simulink model "window_and_fft_test"  (R2012b)
settings: Solver=ode45  StartTime=0.0  StopTime=100000  RelTol=1e-3
values from neighbouring files (symbols this model uses):
  Fs = 640e6    (= 640000000)    [filter_coefficients.m]    (also in filter_design.m; filter_design_getting_order.m)
undefined symbols (not defined in the file or in its folder): get, pfb_coeff_gen_calc, sided, Two, xlipgetpartsetting
undefined symbols (not defined in the file): A_cos, A_sin, B_cos, B_sin, C_cos, C_sin, casper_coef, D_cos, D_sin
libraries: xbsIndex_r4 x7054, casper_library_misc x43, casper_library_delays x25, dspsnks4 x18, dspspect3 x8, dspsigops x4, xps_library x2, xbsReplacements_r4 x2, casper_library_pfbs x2, simulink x1
(part 4 of 85)

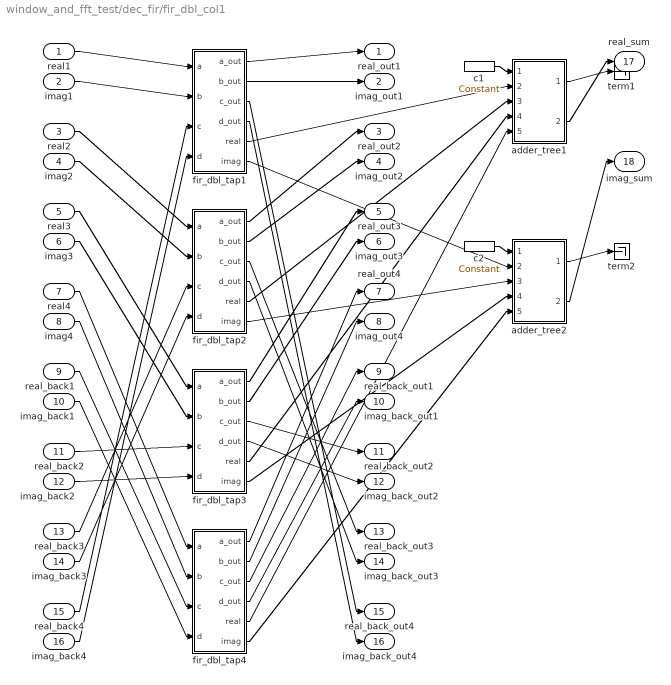
== system window_and_fft_test/dec_fir/fir_dbl_col1 ==
  real1 : Inport
  imag1 : Inport  Port=2
  real2 : Inport  Port=3
  imag2 : Inport  Port=4
  real3 : Inport  Port=5
  imag3 : Inport  Port=6
  real4 : Inport  Port=7
  imag4 : Inport  Port=8
  real_back1 : Inport  Port=9
  imag_back1 : Inport  Port=10
  real_back2 : Inport  Port=11
  imag_back2 : Inport  Port=12
  real_back3 : Inport  Port=13
  imag_back3 : Inport  Port=14
  real_back4 : Inport  Port=15
  imag_back4 : Inport  Port=16
  adder_tree1 : Subsystem  AncestorBlock=casper_library_misc/adder_tree  mask(adder_tree){n_inputs=4, latency=1, adder_imp=DSP48, first_stage_hdl=on}
      mask prompts: n_inputs "Number of Inputs"; latency "Add Latency"; adder_imp "Adder implementation"; first_stage_hdl "Use behavioural HDL for first stage of adders"
      mask help:
      | Sums all inputs using a tree of adds and delays.
      |
      | Number of inputs: The number of inputs to the block to be summed
      | Add latency: The number of clock cycles to perform one addition (affects timing)..
      | Adder implementation: choice of fabric or DSP48E core, or behavioral HDL
      | Use behavioural HDL for first stage of adders: Causes the first stage of adders to be absorbed into DSP blocks if multipliers precede them (Virtex 5). Overrides Adder implementation
      mask init:
      | adder_tree_init(gcb, ...
      |     'n_inputs', n_inputs, ...
      |     'latency', latency, ...
      |     'adder_imp', adder_imp, ...
      |     'first_stage_hdl', first_stage_hdl);
      settings: AttributesFormatString=latency 2
      mask Help: eval('xlWeb(''http://casper.berkeley.edu/wiki/Adder_tree'')')
      mask TypeOptions adder_imp: Behavioral | Fabric | DSP48
  adder_tree2 : Subsystem  AncestorBlock=casper_library_misc/adder_tree  mask(adder_tree){n_inputs=4, latency=1, adder_imp=DSP48, first_stage_hdl=on}
      mask prompts: n_inputs "Number of Inputs"; latency "Add Latency"; adder_imp "Adder implementation"; first_stage_hdl "Use behavioural HDL for first stage of adders"
      mask help:
      | Sums all inputs using a tree of adds and delays.
      |
      | Number of inputs: The number of inputs to the block to be summed
      | Add latency: The number of clock cycles to perform one addition (affects timing)..
      | Adder implementation: choice of fabric or DSP48E core, or behavioral HDL
      | Use behavioural HDL for first stage of adders: Causes the first stage of adders to be absorbed into DSP blocks if multipliers precede them (Virtex 5). Overrides Adder implementation
      mask init:
      | adder_tree_init(gcb, ...
      |     'n_inputs', n_inputs, ...
      |     'latency', latency, ...
      |     'adder_imp', adder_imp, ...
      |     'first_stage_hdl', first_stage_hdl);
      settings: AttributesFormatString=latency 2
      mask Help: eval('xlWeb(''http://casper.berkeley.edu/wiki/Adder_tree'')')
      mask TypeOptions adder_imp: Behavioral | Fabric | DSP48
  c1 : xbsIndex_r4/Constant  const=1  gui_display_data_type=Fixed-point  arith_type=Signed (2's comp)  n_bits=16  bin_pt=14  preci_type=Single  exp_width=8  frac_width=24  explicit_period=on  period=1  equ=P=C  opselect=C  inp2=PCIN>>17  opr=+  inp1=P  carry=CIN  dbl_ovrd=off  block_type=constant
  c2 : xbsIndex_r4/Constant  const=1  gui_display_data_type=Fixed-point  arith_type=Signed (2's comp)  n_bits=16  bin_pt=14  preci_type=Single  exp_width=8  frac_width=24  explicit_period=on  period=1  equ=P=C  opselect=C  inp2=PCIN>>17  opr=+  inp1=P  carry=CIN  dbl_ovrd=off  block_type=constant
  fir_dbl_tap1 : Subsystem  AncestorBlock=casper_library_downconverter/fir_dbl_tap  mask(fir_dbl_tap){factor=0.037109, add_latency=add_latency, mult_latency=mult_latency, coeff_bit_width=coeff_bit_width, coeff_bin_pt=coeff_bin_pt}
      mask prompts: add_latency "Add latency"; mult_latency "Mult latency"; coeff_bit_width "Coefficient bit width"; coeff_bin_pt "Coefficient binary point"
      mask init:
      | fir_dbl_tap_init(gcb, ...
      |     'factor', factor, ...
      |     'add_latency', add_latency, ...
      |     'mult_latency', mult_latency, ...
      |     'coeff_bit_width', coeff_bit_width, ...
      |     'coeff_bin_pt', coeff_bin_pt);
      mask Help: eval('xlWeb(''http://casper.berkeley.edu/wiki/Fir_dbl_tap'')')
  fir_dbl_tap2 : Subsystem  AncestorBlock=casper_library_downconverter/fir_dbl_tap  mask(fir_dbl_tap){factor=0.023207, add_latency=add_latency, mult_latency=mult_latency, coeff_bit_width=coeff_bit_width, coeff_bin_pt=coeff_bin_pt}
      mask prompts: add_latency "Add latency"; mult_latency "Mult latency"; coeff_bit_width "Coefficient bit width"; coeff_bin_pt "Coefficient binary point"
      mask init: same as window_and_fft_test/dec_fir/fir_dbl_col1/fir_dbl_tap1
      mask Help: eval('xlWeb(''http://casper.berkeley.edu/wiki/Fir_dbl_tap'')')
  fir_dbl_tap3 : Subsystem  AncestorBlock=casper_library_downconverter/fir_dbl_tap  mask(fir_dbl_tap){factor=0.012354, add_latency=add_latency, mult_latency=mult_latency, coeff_bit_width=coeff_bit_width, coeff_bin_pt=coeff_bin_pt}
      mask prompts: add_latency "Add latency"; mult_latency "Mult latency"; coeff_bit_width "Coefficient bit width"; coeff_bin_pt "Coefficient binary point"
      mask init: same as window_and_fft_test/dec_fir/fir_dbl_col1/fir_dbl_tap1
      mask Help: eval('xlWeb(''http://casper.berkeley.edu/wiki/Fir_dbl_tap'')')
  fir_dbl_tap4 : Subsystem  AncestorBlock=casper_library_downconverter/fir_dbl_tap  mask(fir_dbl_tap){factor=0.0056253, add_latency=add_latency, mult_latency=mult_latency, coeff_bit_width=coeff_bit_width, coeff_bin_pt=coeff_bin_pt}
      mask prompts: add_latency "Add latency"; mult_latency "Mult latency"; coeff_bit_width "Coefficient bit width"; coeff_bin_pt "Coefficient binary point"
      mask init: same as window_and_fft_test/dec_fir/fir_dbl_col1/fir_dbl_tap1
      mask Help: eval('xlWeb(''http://casper.berkeley.edu/wiki/Fir_dbl_tap'')')
  term1 : Terminator
  term2 : Terminator
  real_out1 : Outport
  imag_out1 : Outport  Port=2
  real_out2 : Outport  Port=3
  imag_out2 : Outport  Port=4
  real_out3 : Outport  Port=5
  imag_out3 : Outport  Port=6
  real_out4 : Outport  Port=7
  imag_out4 : Outport  Port=8
  real_back_out1 : Outport  Port=9
  imag_back_out1 : Outport  Port=10
  real_back_out2 : Outport  Port=11
  imag_back_out2 : Outport  Port=12
  real_back_out3 : Outport  Port=13
  imag_back_out3 : Outport  Port=14
  real_back_out4 : Outport  Port=15
  imag_back_out4 : Outport  Port=16
  real_sum : Outport  Port=17
  imag_sum : Outport  Port=18
  wires:
  adder_tree1/1(sync_out) -> term1/1
  adder_tree2/1(sync_out) -> term2/1
  c1/1 -> adder_tree1/1(sync)
  c2/1 -> adder_tree2/1(sync)
  adder_tree1/2(dout) -> real_sum/1
  adder_tree2/2(dout) -> imag_sum/1
  real1/1 -> fir_dbl_tap1/1(a)
  imag1/1 -> fir_dbl_tap1/2(b)
  real_back4/1 -> fir_dbl_tap1/3(c)
  imag_back4/1 -> fir_dbl_tap1/4(d)
  fir_dbl_tap1/1(a_out) -> real_out1/1
  fir_dbl_tap1/2(b_out) -> imag_out1/1
  fir_dbl_tap1/3(c_out) -> real_back_out4/1
  fir_dbl_tap1/4(d_out) -> imag_back_out4/1
  fir_dbl_tap1/5(real) -> adder_tree1/2(din1)
  fir_dbl_tap1/6(imag) -> adder_tree2/2(din1)
  real2/1 -> fir_dbl_tap2/1(a)
  imag2/1 -> fir_dbl_tap2/2(b)
  real_back3/1 -> fir_dbl_tap2/3(c)
  imag_back3/1 -> fir_dbl_tap2/4(d)
  fir_dbl_tap2/1(a_out) -> real_out2/1
  fir_dbl_tap2/2(b_out) -> imag_out2/1
  fir_dbl_tap2/3(c_out) -> real_back_out3/1
  fir_dbl_tap2/4(d_out) -> imag_back_out3/1
  fir_dbl_tap2/5(real) -> adder_tree1/3(din2)
  fir_dbl_tap2/6(imag) -> adder_tree2/3(din2)
  real3/1 -> fir_dbl_tap3/1(a)
  imag3/1 -> fir_dbl_tap3/2(b)
  real_back2/1 -> fir_dbl_tap3/3(c)
  imag_back2/1 -> fir_dbl_tap3/4(d)
  fir_dbl_tap3/1(a_out) -> real_out3/1
  fir_dbl_tap3/2(b_out) -> imag_out3/1
  fir_dbl_tap3/3(c_out) -> real_back_out2/1
  fir_dbl_tap3/4(d_out) -> imag_back_out2/1
  fir_dbl_tap3/5(real) -> adder_tree1/4(din3)
  fir_dbl_tap3/6(imag) -> adder_tree2/4(din3)
  real4/1 -> fir_dbl_tap4/1(a)
  imag4/1 -> fir_dbl_tap4/2(b)
  real_back1/1 -> fir_dbl_tap4/3(c)
  imag_back1/1 -> fir_dbl_tap4/4(d)
  fir_dbl_tap4/1(a_out) -> real_out4/1
  fir_dbl_tap4/2(b_out) -> imag_out4/1
  fir_dbl_tap4/3(c_out) -> real_back_out1/1
  fir_dbl_tap4/4(d_out) -> imag_back_out1/1
  fir_dbl_tap4/5(real) -> adder_tree1/5(din4)
  fir_dbl_tap4/6(imag) -> adder_tree2/5(din4)

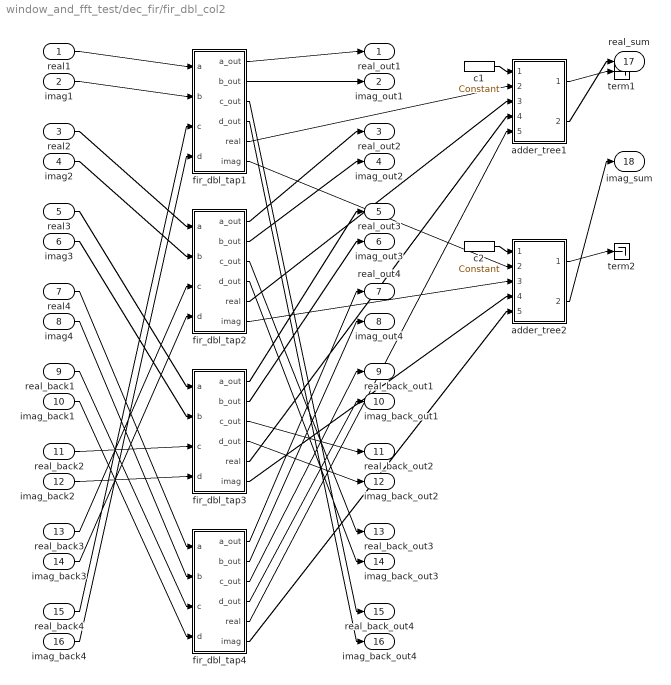
== system window_and_fft_test/dec_fir/fir_dbl_col2 ==
  real1 : Inport
  imag1 : Inport  Port=2
  real2 : Inport  Port=3
  imag2 : Inport  Port=4
  real3 : Inport  Port=5
  imag3 : Inport  Port=6
  real4 : Inport  Port=7
  imag4 : Inport  Port=8
  real_back1 : Inport  Port=9
  imag_back1 : Inport  Port=10
  real_back2 : Inport  Port=11
  imag_back2 : Inport  Port=12
  real_back3 : Inport  Port=13
  imag_back3 : Inport  Port=14
  real_back4 : Inport  Port=15
  imag_back4 : Inport  Port=16
  adder_tree1 : Subsystem  AncestorBlock=casper_library_misc/adder_tree  mask(adder_tree){n_inputs=4, latency=1, adder_imp=DSP48, first_stage_hdl=on}
      mask prompts: n_inputs "Number of Inputs"; latency "Add Latency"; adder_imp "Adder implementation"; first_stage_hdl "Use behavioural HDL for first stage of adders"
      mask help:
      | Sums all inputs using a tree of adds and delays.
      |
      | Number of inputs: The number of inputs to the block to be summed
      | Add latency: The number of clock cycles to perform one addition (affects timing)..
      | Adder implementation: choice of fabric or DSP48E core, or behavioral HDL
      | Use behavioural HDL for first stage of adders: Causes the first stage of adders to be absorbed into DSP blocks if multipliers precede them (Virtex 5). Overrides Adder implementation
      mask init:
      | adder_tree_init(gcb, ...
      |     'n_inputs', n_inputs, ...
      |     'latency', latency, ...
      |     'adder_imp', adder_imp, ...
      |     'first_stage_hdl', first_stage_hdl);
      settings: AttributesFormatString=latency 2
      mask Help: eval('xlWeb(''http://casper.berkeley.edu/wiki/Adder_tree'')')
      mask TypeOptions adder_imp: Behavioral | Fabric | DSP48
  adder_tree2 : Subsystem  AncestorBlock=casper_library_misc/adder_tree  mask(adder_tree){n_inputs=4, latency=1, adder_imp=DSP48, first_stage_hdl=on}
      mask prompts: n_inputs "Number of Inputs"; latency "Add Latency"; adder_imp "Adder implementation"; first_stage_hdl "Use behavioural HDL for first stage of adders"
      mask help:
      | Sums all inputs using a tree of adds and delays.
      |
      | Number of inputs: The number of inputs to the block to be summed
      | Add latency: The number of clock cycles to perform one addition (affects timing)..
      | Adder implementation: choice of fabric or DSP48E core, or behavioral HDL
      | Use behavioural HDL for first stage of adders: Causes the first stage of adders to be absorbed into DSP blocks if multipliers precede them (Virtex 5). Overrides Adder implementation
      mask init:
      | adder_tree_init(gcb, ...
      |     'n_inputs', n_inputs, ...
      |     'latency', latency, ...
      |     'adder_imp', adder_imp, ...
      |     'first_stage_hdl', first_stage_hdl);
      settings: AttributesFormatString=latency 2
      mask Help: eval('xlWeb(''http://casper.berkeley.edu/wiki/Adder_tree'')')
      mask TypeOptions adder_imp: Behavioral | Fabric | DSP48
  c1 : xbsIndex_r4/Constant  const=1  gui_display_data_type=Fixed-point  arith_type=Signed (2's comp)  n_bits=16  bin_pt=14  preci_type=Single  exp_width=8  frac_width=24  explicit_period=on  period=1  equ=P=C  opselect=C  inp2=PCIN>>17  opr=+  inp1=P  carry=CIN  dbl_ovrd=off  block_type=constant
  c2 : xbsIndex_r4/Constant  const=1  gui_display_data_type=Fixed-point  arith_type=Signed (2's comp)  n_bits=16  bin_pt=14  preci_type=Single  exp_width=8  frac_width=24  explicit_period=on  period=1  equ=P=C  opselect=C  inp2=PCIN>>17  opr=+  inp1=P  carry=CIN  dbl_ovrd=off  block_type=constant
  fir_dbl_tap1 : Subsystem  AncestorBlock=casper_library_downconverter/fir_dbl_tap  mask(fir_dbl_tap){factor=0.08556, add_latency=add_latency, mult_latency=mult_latency, coeff_bit_width=coeff_bit_width, coeff_bin_pt=coeff_bin_pt}
      mask prompts: add_latency "Add latency"; mult_latency "Mult latency"; coeff_bit_width "Coefficient bit width"; coeff_bin_pt "Coefficient binary point"
      mask init: same as window_and_fft_test/dec_fir/fir_dbl_col1/fir_dbl_tap1
      mask Help: eval('xlWeb(''http://casper.berkeley.edu/wiki/Fir_dbl_tap'')')
  fir_dbl_tap2 : Subsystem  AncestorBlock=casper_library_downconverter/fir_dbl_tap  mask(fir_dbl_tap){factor=0.079092, add_latency=add_latency, mult_latency=mult_latency, coeff_bit_width=coeff_bit_width, coeff_bin_pt=coeff_bin_pt}
      mask prompts: add_latency "Add latency"; mult_latency "Mult latency"; coeff_bit_width "Coefficient bit width"; coeff_bin_pt "Coefficient binary point"
      mask init: same as window_and_fft_test/dec_fir/fir_dbl_col1/fir_dbl_tap1
      mask Help: eval('xlWeb(''http://casper.berkeley.edu/wiki/Fir_dbl_tap'')')
  fir_dbl_tap3 : Subsystem  AncestorBlock=casper_library_downconverter/fir_dbl_tap  mask(fir_dbl_tap){factor=0.067391, add_latency=add_latency, mult_latency=mult_latency, coeff_bit_width=coeff_bit_width, coeff_bin_pt=coeff_bin_pt}
      mask prompts: add_latency "Add latency"; mult_latency "Mult latency"; coeff_bit_width "Coefficient bit width"; coeff_bin_pt "Coefficient binary point"
      mask init: same as window_and_fft_test/dec_fir/fir_dbl_col1/fir_dbl_tap1
      mask Help: eval('xlWeb(''http://casper.berkeley.edu/wiki/Fir_dbl_tap'')')
  fir_dbl_tap4 : Subsystem  AncestorBlock=casper_library_downconverter/fir_dbl_tap  mask(fir_dbl_tap){factor=0.052572, add_latency=add_latency, mult_latency=mult_latency, coeff_bit_width=coeff_bit_width, coeff_bin_pt=coeff_bin_pt}
      mask prompts: add_latency "Add latency"; mult_latency "Mult latency"; coeff_bit_width "Coefficient bit width"; coeff_bin_pt "Coefficient binary point"
      mask init: same as window_and_fft_test/dec_fir/fir_dbl_col1/fir_dbl_tap1
      mask Help: eval('xlWeb(''http://casper.berkeley.edu/wiki/Fir_dbl_tap'')')
  term1 : Terminator
  term2 : Terminator
  real_out1 : Outport
  imag_out1 : Outport  Port=2
  real_out2 : Outport  Port=3
  imag_out2 : Outport  Port=4
  real_out3 : Outport  Port=5
  imag_out3 : Outport  Port=6
  real_out4 : Outport  Port=7
  imag_out4 : Outport  Port=8
  real_back_out1 : Outport  Port=9
  imag_back_out1 : Outport  Port=10
  real_back_out2 : Outport  Port=11
  imag_back_out2 : Outport  Port=12
  real_back_out3 : Outport  Port=13
  imag_back_out3 : Outport  Port=14
  real_back_out4 : Outport  Port=15
  imag_back_out4 : Outport  Port=16
  real_sum : Outport  Port=17
  imag_sum : Outport  Port=18
  wires:
  adder_tree1/1(sync_out) -> term1/1
  adder_tree2/1(sync_out) -> term2/1
  c1/1 -> adder_tree1/1(sync)
  c2/1 -> adder_tree2/1(sync)
  adder_tree1/2(dout) -> real_sum/1
  adder_tree2/2(dout) -> imag_sum/1
  real1/1 -> fir_dbl_tap1/1(a)
  imag1/1 -> fir_dbl_tap1/2(b)
  real_back4/1 -> fir_dbl_tap1/3(c)
  imag_back4/1 -> fir_dbl_tap1/4(d)
  fir_dbl_tap1/1(a_out) -> real_out1/1
  fir_dbl_tap1/2(b_out) -> imag_out1/1
  fir_dbl_tap1/3(c_out) -> real_back_out4/1
  fir_dbl_tap1/4(d_out) -> imag_back_out4/1
  fir_dbl_tap1/5(real) -> adder_tree1/2(din1)
  fir_dbl_tap1/6(imag) -> adder_tree2/2(din1)
  real2/1 -> fir_dbl_tap2/1(a)
  imag2/1 -> fir_dbl_tap2/2(b)
  real_back3/1 -> fir_dbl_tap2/3(c)
  imag_back3/1 -> fir_dbl_tap2/4(d)
  fir_dbl_tap2/1(a_out) -> real_out2/1
  fir_dbl_tap2/2(b_out) -> imag_out2/1
  fir_dbl_tap2/3(c_out) -> real_back_out3/1
  fir_dbl_tap2/4(d_out) -> imag_back_out3/1
  fir_dbl_tap2/5(real) -> adder_tree1/3(din2)
  fir_dbl_tap2/6(imag) -> adder_tree2/3(din2)
  real3/1 -> fir_dbl_tap3/1(a)
  imag3/1 -> fir_dbl_tap3/2(b)
  real_back2/1 -> fir_dbl_tap3/3(c)
  imag_back2/1 -> fir_dbl_tap3/4(d)
  fir_dbl_tap3/1(a_out) -> real_out3/1
  fir_dbl_tap3/2(b_out) -> imag_out3/1
  fir_dbl_tap3/3(c_out) -> real_back_out2/1
  fir_dbl_tap3/4(d_out) -> imag_back_out2/1
  fir_dbl_tap3/5(real) -> adder_tree1/4(din3)
  fir_dbl_tap3/6(imag) -> adder_tree2/4(din3)
  real4/1 -> fir_dbl_tap4/1(a)
  imag4/1 -> fir_dbl_tap4/2(b)
  real_back1/1 -> fir_dbl_tap4/3(c)
  imag_back1/1 -> fir_dbl_tap4/4(d)
  fir_dbl_tap4/1(a_out) -> real_out4/1
  fir_dbl_tap4/2(b_out) -> imag_out4/1
  fir_dbl_tap4/3(c_out) -> real_back_out1/1
  fir_dbl_tap4/4(d_out) -> imag_back_out1/1
  fir_dbl_tap4/5(real) -> adder_tree1/5(din4)
  fir_dbl_tap4/6(imag) -> adder_tree2/5(din4)

== system window_and_fft_test/dec_fir/imag_sum ==
  sync : Inport
  din1 : Inport  Port=2
  din2 : Inport  Port=3
  addr1 : xbsIndex_r4/AddSub  mode=Addition  use_carryin=off  use_carryout=off  en=off  latency=1  precision=Full  arith_type=Unsigned  n_bits=16  bin_pt=14  quantization=Truncate  overflow=Wrap  dbl_ovrd=off  use_behavioral_HDL=off  hw_selection=DSP48  pipelined=on  use_rpm=on  block_type=addsub
  sync_delay : xbsIndex_r4/Delay  rst=off  infoeditControl=Selection of Reset will increase slice count due to use of real FFs and instead of SRLs  en=off  latency=1  dbl_ovrd=off  reg_retiming=on  block_type=delay
      settings: block_version=11.4
  sync_out : Outport
  dout : Outport  Port=2
  wires:
  sync/1 -> sync_delay/1
  sync_delay/1 -> sync_out/1
  din1/1 -> addr1/1
  din2/1 -> addr1/2
  addr1/1 -> dout/1

== system window_and_fft_test/dec_fir/real_sum ==
  sync : Inport
  din1 : Inport  Port=2
  din2 : Inport  Port=3
  addr1 : xbsIndex_r4/AddSub  mode=Addition  use_carryin=off  use_carryout=off  en=off  latency=1  precision=Full  arith_type=Unsigned  n_bits=16  bin_pt=14  quantization=Truncate  overflow=Wrap  dbl_ovrd=off  use_behavioral_HDL=off  hw_selection=DSP48  pipelined=on  use_rpm=on  block_type=addsub
  sync_delay : xbsIndex_r4/Delay  rst=off  infoeditControl=Selection of Reset will increase slice count due to use of real FFs and instead of SRLs  en=off  latency=1  dbl_ovrd=off  reg_retiming=on  block_type=delay
      settings: block_version=11.4
  sync_out : Outport
  dout : Outport  Port=2
  wires:
  sync/1 -> sync_delay/1
  sync_delay/1 -> sync_out/1
  din1/1 -> addr1/1
  din2/1 -> addr1/2
  addr1/1 -> dout/1

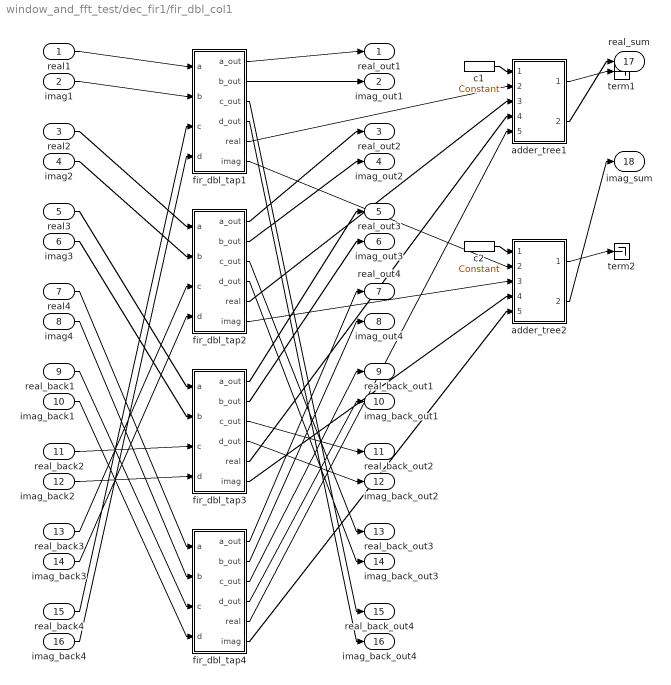
== system window_and_fft_test/dec_fir1/fir_dbl_col1 ==
  real1 : Inport
  imag1 : Inport  Port=2
  real2 : Inport  Port=3
  imag2 : Inport  Port=4
  real3 : Inport  Port=5
  imag3 : Inport  Port=6
  real4 : Inport  Port=7
  imag4 : Inport  Port=8
  real_back1 : Inport  Port=9
  imag_back1 : Inport  Port=10
  real_back2 : Inport  Port=11
  imag_back2 : Inport  Port=12
  real_back3 : Inport  Port=13
  imag_back3 : Inport  Port=14
  real_back4 : Inport  Port=15
  imag_back4 : Inport  Port=16
  adder_tree1 : Subsystem  AncestorBlock=casper_library_misc/adder_tree  mask(adder_tree){n_inputs=4, latency=1, adder_imp=DSP48, first_stage_hdl=on}
      mask prompts: n_inputs "Number of Inputs"; latency "Add Latency"; adder_imp "Adder implementation"; first_stage_hdl "Use behavioural HDL for first stage of adders"
      mask help:
      | Sums all inputs using a tree of adds and delays.
      |
      | Number of inputs: The number of inputs to the block to be summed
      | Add latency: The number of clock cycles to perform one addition (affects timing)..
      | Adder implementation: choice of fabric or DSP48E core, or behavioral HDL
      | Use behavioural HDL for first stage of adders: Causes the first stage of adders to be absorbed into DSP blocks if multipliers precede them (Virtex 5). Overrides Adder implementation
      mask init:
      | adder_tree_init(gcb, ...
      |     'n_inputs', n_inputs, ...
      |     'latency', latency, ...
      |     'adder_imp', adder_imp, ...
      |     'first_stage_hdl', first_stage_hdl);
      settings: AttributesFormatString=latency 2
      mask Help: eval('xlWeb(''http://casper.berkeley.edu/wiki/Adder_tree'')')
      mask TypeOptions adder_imp: Behavioral | Fabric | DSP48
  adder_tree2 : Subsystem  AncestorBlock=casper_library_misc/adder_tree  mask(adder_tree){n_inputs=4, latency=1, adder_imp=DSP48, first_stage_hdl=on}
      mask prompts: n_inputs "Number of Inputs"; latency "Add Latency"; adder_imp "Adder implementation"; first_stage_hdl "Use behavioural HDL for first stage of adders"
      mask help:
      | Sums all inputs using a tree of adds and delays.
      |
      | Number of inputs: The number of inputs to the block to be summed
      | Add latency: The number of clock cycles to perform one addition (affects timing)..
      | Adder implementation: choice of fabric or DSP48E core, or behavioral HDL
      | Use behavioural HDL for first stage of adders: Causes the first stage of adders to be absorbed into DSP blocks if multipliers precede them (Virtex 5). Overrides Adder implementation
      mask init:
      | adder_tree_init(gcb, ...
      |     'n_inputs', n_inputs, ...
      |     'latency', latency, ...
      |     'adder_imp', adder_imp, ...
      |     'first_stage_hdl', first_stage_hdl);
      settings: AttributesFormatString=latency 2
      mask Help: eval('xlWeb(''http://casper.berkeley.edu/wiki/Adder_tree'')')
      mask TypeOptions adder_imp: Behavioral | Fabric | DSP48
  c1 : xbsIndex_r4/Constant  const=1  gui_display_data_type=Fixed-point  arith_type=Signed (2's comp)  n_bits=16  bin_pt=14  preci_type=Single  exp_width=8  frac_width=24  explicit_period=on  period=1  equ=P=C  opselect=C  inp2=PCIN>>17  opr=+  inp1=P  carry=CIN  dbl_ovrd=off  block_type=constant
  c2 : xbsIndex_r4/Constant  const=1  gui_display_data_type=Fixed-point  arith_type=Signed (2's comp)  n_bits=16  bin_pt=14  preci_type=Single  exp_width=8  frac_width=24  explicit_period=on  period=1  equ=P=C  opselect=C  inp2=PCIN>>17  opr=+  inp1=P  carry=CIN  dbl_ovrd=off  block_type=constant
  fir_dbl_tap1 : Subsystem  AncestorBlock=casper_library_downconverter/fir_dbl_tap  mask(fir_dbl_tap){factor=0.037109, add_latency=add_latency, mult_latency=mult_latency, coeff_bit_width=coeff_bit_width, coeff_bin_pt=coeff_bin_pt}
      mask prompts: add_latency "Add latency"; mult_latency "Mult latency"; coeff_bit_width "Coefficient bit width"; coeff_bin_pt "Coefficient binary point"
      mask init: same as window_and_fft_test/dec_fir/fir_dbl_col1/fir_dbl_tap1
      mask Help: eval('xlWeb(''http://casper.berkeley.edu/wiki/Fir_dbl_tap'')')
  fir_dbl_tap2 : Subsystem  AncestorBlock=casper_library_downconverter/fir_dbl_tap  mask(fir_dbl_tap){factor=0.023207, add_latency=add_latency, mult_latency=mult_latency, coeff_bit_width=coeff_bit_width, coeff_bin_pt=coeff_bin_pt}
      mask prompts: add_latency "Add latency"; mult_latency "Mult latency"; coeff_bit_width "Coefficient bit width"; coeff_bin_pt "Coefficient binary point"
      mask init: same as window_and_fft_test/dec_fir/fir_dbl_col1/fir_dbl_tap1
      mask Help: eval('xlWeb(''http://casper.berkeley.edu/wiki/Fir_dbl_tap'')')
  fir_dbl_tap3 : Subsystem  AncestorBlock=casper_library_downconverter/fir_dbl_tap  mask(fir_dbl_tap){factor=0.012354, add_latency=add_latency, mult_latency=mult_latency, coeff_bit_width=coeff_bit_width, coeff_bin_pt=coeff_bin_pt}
      mask prompts: add_latency "Add latency"; mult_latency "Mult latency"; coeff_bit_width "Coefficient bit width"; coeff_bin_pt "Coefficient binary point"
      mask init: same as window_and_fft_test/dec_fir/fir_dbl_col1/fir_dbl_tap1
      mask Help: eval('xlWeb(''http://casper.berkeley.edu/wiki/Fir_dbl_tap'')')
  fir_dbl_tap4 : Subsystem  AncestorBlock=casper_library_downconverter/fir_dbl_tap  mask(fir_dbl_tap){factor=0.0056253, add_latency=add_latency, mult_latency=mult_latency, coeff_bit_width=coeff_bit_width, coeff_bin_pt=coeff_bin_pt}
      mask prompts: add_latency "Add latency"; mult_latency "Mult latency"; coeff_bit_width "Coefficient bit width"; coeff_bin_pt "Coefficient binary point"
      mask init: same as window_and_fft_test/dec_fir/fir_dbl_col1/fir_dbl_tap1
      mask Help: eval('xlWeb(''http://casper.berkeley.edu/wiki/Fir_dbl_tap'')')
  term1 : Terminator
  term2 : Terminator
  real_out1 : Outport
  imag_out1 : Outport  Port=2
  real_out2 : Outport  Port=3
  imag_out2 : Outport  Port=4
  real_out3 : Outport  Port=5
  imag_out3 : Outport  Port=6
  real_out4 : Outport  Port=7
  imag_out4 : Outport  Port=8
  real_back_out1 : Outport  Port=9
  imag_back_out1 : Outport  Port=10
  real_back_out2 : Outport  Port=11
  imag_back_out2 : Outport  Port=12
  real_back_out3 : Outport  Port=13
  imag_back_out3 : Outport  Port=14
  real_back_out4 : Outport  Port=15
  imag_back_out4 : Outport  Port=16
  real_sum : Outport  Port=17
  imag_sum : Outport  Port=18
  wires:
  adder_tree1/1(sync_out) -> term1/1
  adder_tree2/1(sync_out) -> term2/1
  c1/1 -> adder_tree1/1(sync)
  c2/1 -> adder_tree2/1(sync)
  adder_tree1/2(dout) -> real_sum/1
  adder_tree2/2(dout) -> imag_sum/1
  real1/1 -> fir_dbl_tap1/1(a)
  imag1/1 -> fir_dbl_tap1/2(b)
  real_back4/1 -> fir_dbl_tap1/3(c)
  imag_back4/1 -> fir_dbl_tap1/4(d)
  fir_dbl_tap1/1(a_out) -> real_out1/1
  fir_dbl_tap1/2(b_out) -> imag_out1/1
  fir_dbl_tap1/3(c_out) -> real_back_out4/1
  fir_dbl_tap1/4(d_out) -> imag_back_out4/1
  fir_dbl_tap1/5(real) -> adder_tree1/2(din1)
  fir_dbl_tap1/6(imag) -> adder_tree2/2(din1)
  real2/1 -> fir_dbl_tap2/1(a)
  imag2/1 -> fir_dbl_tap2/2(b)
  real_back3/1 -> fir_dbl_tap2/3(c)
  imag_back3/1 -> fir_dbl_tap2/4(d)
  fir_dbl_tap2/1(a_out) -> real_out2/1
  fir_dbl_tap2/2(b_out) -> imag_out2/1
  fir_dbl_tap2/3(c_out) -> real_back_out3/1
  fir_dbl_tap2/4(d_out) -> imag_back_out3/1
  fir_dbl_tap2/5(real) -> adder_tree1/3(din2)
  fir_dbl_tap2/6(imag) -> adder_tree2/3(din2)
  real3/1 -> fir_dbl_tap3/1(a)
  imag3/1 -> fir_dbl_tap3/2(b)
  real_back2/1 -> fir_dbl_tap3/3(c)
  imag_back2/1 -> fir_dbl_tap3/4(d)
  fir_dbl_tap3/1(a_out) -> real_out3/1
  fir_dbl_tap3/2(b_out) -> imag_out3/1
  fir_dbl_tap3/3(c_out) -> real_back_out2/1
  fir_dbl_tap3/4(d_out) -> imag_back_out2/1
  fir_dbl_tap3/5(real) -> adder_tree1/4(din3)
  fir_dbl_tap3/6(imag) -> adder_tree2/4(din3)
  real4/1 -> fir_dbl_tap4/1(a)
  imag4/1 -> fir_dbl_tap4/2(b)
  real_back1/1 -> fir_dbl_tap4/3(c)
  imag_back1/1 -> fir_dbl_tap4/4(d)
  fir_dbl_tap4/1(a_out) -> real_out4/1
  fir_dbl_tap4/2(b_out) -> imag_out4/1
  fir_dbl_tap4/3(c_out) -> real_back_out1/1
  fir_dbl_tap4/4(d_out) -> imag_back_out1/1
  fir_dbl_tap4/5(real) -> adder_tree1/5(din4)
  fir_dbl_tap4/6(imag) -> adder_tree2/5(din4)

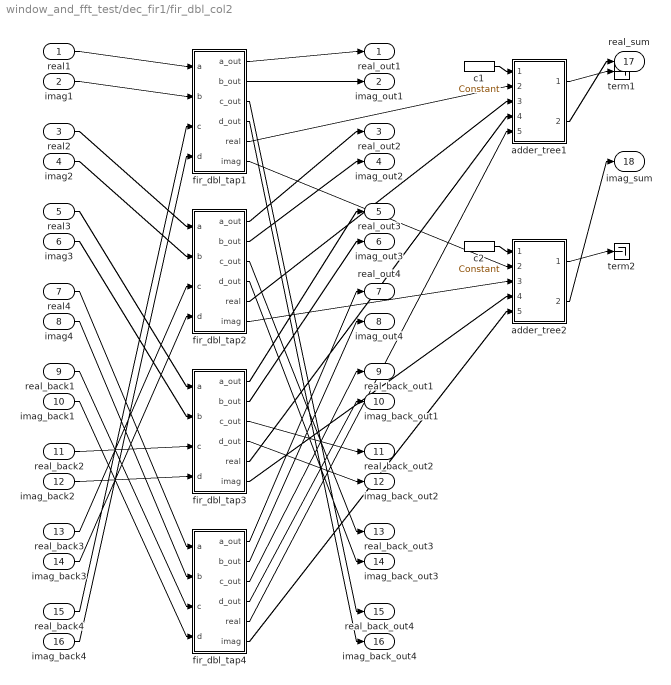
== system window_and_fft_test/dec_fir1/fir_dbl_col2 ==
  real1 : Inport
  imag1 : Inport  Port=2
  real2 : Inport  Port=3
  imag2 : Inport  Port=4
  real3 : Inport  Port=5
  imag3 : Inport  Port=6
  real4 : Inport  Port=7
  imag4 : Inport  Port=8
  real_back1 : Inport  Port=9
  imag_back1 : Inport  Port=10
  real_back2 : Inport  Port=11
  imag_back2 : Inport  Port=12
  real_back3 : Inport  Port=13
  imag_back3 : Inport  Port=14
  real_back4 : Inport  Port=15
  imag_back4 : Inport  Port=16
  adder_tree1 : Subsystem  AncestorBlock=casper_library_misc/adder_tree  mask(adder_tree){n_inputs=4, latency=1, adder_imp=DSP48, first_stage_hdl=on}
      mask prompts: n_inputs "Number of Inputs"; latency "Add Latency"; adder_imp "Adder implementation"; first_stage_hdl "Use behavioural HDL for first stage of adders"
      mask help:
      | Sums all inputs using a tree of adds and delays.
      |
      | Number of inputs: The number of inputs to the block to be summed
      | Add latency: The number of clock cycles to perform one addition (affects timing)..
      | Adder implementation: choice of fabric or DSP48E core, or behavioral HDL
      | Use behavioural HDL for first stage of adders: Causes the first stage of adders to be absorbed into DSP blocks if multipliers precede them (Virtex 5). Overrides Adder implementation
      mask init:
      | adder_tree_init(gcb, ...
      |     'n_inputs', n_inputs, ...
      |     'latency', latency, ...
      |     'adder_imp', adder_imp, ...
      |     'first_stage_hdl', first_stage_hdl);
      settings: AttributesFormatString=latency 2
      mask Help: eval('xlWeb(''http://casper.berkeley.edu/wiki/Adder_tree'')')
      mask TypeOptions adder_imp: Behavioral | Fabric | DSP48
  adder_tree2 : Subsystem  AncestorBlock=casper_library_misc/adder_tree  mask(adder_tree){n_inputs=4, latency=1, adder_imp=DSP48, first_stage_hdl=on}
      mask prompts: n_inputs "Number of Inputs"; latency "Add Latency"; adder_imp "Adder implementation"; first_stage_hdl "Use behavioural HDL for first stage of adders"
      mask help:
      | Sums all inputs using a tree of adds and delays.
      |
      | Number of inputs: The number of inputs to the block to be summed
      | Add latency: The number of clock cycles to perform one addition (affects timing)..
      | Adder implementation: choice of fabric or DSP48E core, or behavioral HDL
      | Use behavioural HDL for first stage of adders: Causes the first stage of adders to be absorbed into DSP blocks if multipliers precede them (Virtex 5). Overrides Adder implementation
      mask init:
      | adder_tree_init(gcb, ...
      |     'n_inputs', n_inputs, ...
      |     'latency', latency, ...
      |     'adder_imp', adder_imp, ...
      |     'first_stage_hdl', first_stage_hdl);
      settings: AttributesFormatString=latency 2
      mask Help: eval('xlWeb(''http://casper.berkeley.edu/wiki/Adder_tree'')')
      mask TypeOptions adder_imp: Behavioral | Fabric | DSP48
  c1 : xbsIndex_r4/Constant  const=1  gui_display_data_type=Fixed-point  arith_type=Signed (2's comp)  n_bits=16  bin_pt=14  preci_type=Single  exp_width=8  frac_width=24  explicit_period=on  period=1  equ=P=C  opselect=C  inp2=PCIN>>17  opr=+  inp1=P  carry=CIN  dbl_ovrd=off  block_type=constant
  c2 : xbsIndex_r4/Constant  const=1  gui_display_data_type=Fixed-point  arith_type=Signed (2's comp)  n_bits=16  bin_pt=14  preci_type=Single  exp_width=8  frac_width=24  explicit_period=on  period=1  equ=P=C  opselect=C  inp2=PCIN>>17  opr=+  inp1=P  carry=CIN  dbl_ovrd=off  block_type=constant
  fir_dbl_tap1 : Subsystem  AncestorBlock=casper_library_downconverter/fir_dbl_tap  mask(fir_dbl_tap){factor=0.08556, add_latency=add_latency, mult_latency=mult_latency, coeff_bit_width=coeff_bit_width, coeff_bin_pt=coeff_bin_pt}
      mask prompts: add_latency "Add latency"; mult_latency "Mult latency"; coeff_bit_width "Coefficient bit width"; coeff_bin_pt "Coefficient binary point"
      mask init: same as window_and_fft_test/dec_fir/fir_dbl_col1/fir_dbl_tap1
      mask Help: eval('xlWeb(''http://casper.berkeley.edu/wiki/Fir_dbl_tap'')')
  fir_dbl_tap2 : Subsystem  AncestorBlock=casper_library_downconverter/fir_dbl_tap  mask(fir_dbl_tap){factor=0.079092, add_latency=add_latency, mult_latency=mult_latency, coeff_bit_width=coeff_bit_width, coeff_bin_pt=coeff_bin_pt}
      mask prompts: add_latency "Add latency"; mult_latency "Mult latency"; coeff_bit_width "Coefficient bit width"; coeff_bin_pt "Coefficient binary point"
      mask init: same as window_and_fft_test/dec_fir/fir_dbl_col1/fir_dbl_tap1
      mask Help: eval('xlWeb(''http://casper.berkeley.edu/wiki/Fir_dbl_tap'')')
  fir_dbl_tap3 : Subsystem  AncestorBlock=casper_library_downconverter/fir_dbl_tap  mask(fir_dbl_tap){factor=0.067391, add_latency=add_latency, mult_latency=mult_latency, coeff_bit_width=coeff_bit_width, coeff_bin_pt=coeff_bin_pt}
      mask prompts: add_latency "Add latency"; mult_latency "Mult latency"; coeff_bit_width "Coefficient bit width"; coeff_bin_pt "Coefficient binary point"
      mask init: same as window_and_fft_test/dec_fir/fir_dbl_col1/fir_dbl_tap1
      mask Help: eval('xlWeb(''http://casper.berkeley.edu/wiki/Fir_dbl_tap'')')
  fir_dbl_tap4 : Subsystem  AncestorBlock=casper_library_downconverter/fir_dbl_tap  mask(fir_dbl_tap){factor=0.052572, add_latency=add_latency, mult_latency=mult_latency, coeff_bit_width=coeff_bit_width, coeff_bin_pt=coeff_bin_pt}
      mask prompts: add_latency "Add latency"; mult_latency "Mult latency"; coeff_bit_width "Coefficient bit width"; coeff_bin_pt "Coefficient binary point"
      mask init: same as window_and_fft_test/dec_fir/fir_dbl_col1/fir_dbl_tap1
      mask Help: eval('xlWeb(''http://casper.berkeley.edu/wiki/Fir_dbl_tap'')')
  term1 : Terminator
  term2 : Terminator
  real_out1 : Outport
  imag_out1 : Outport  Port=2
  real_out2 : Outport  Port=3
  imag_out2 : Outport  Port=4
  real_out3 : Outport  Port=5
  imag_out3 : Outport  Port=6
  real_out4 : Outport  Port=7
  imag_out4 : Outport  Port=8
  real_back_out1 : Outport  Port=9
  imag_back_out1 : Outport  Port=10
  real_back_out2 : Outport  Port=11
  imag_back_out2 : Outport  Port=12
  real_back_out3 : Outport  Port=13
  imag_back_out3 : Outport  Port=14
  real_back_out4 : Outport  Port=15
  imag_back_out4 : Outport  Port=16
  real_sum : Outport  Port=17
  imag_sum : Outport  Port=18
  wires:
  adder_tree1/1(sync_out) -> term1/1
  adder_tree2/1(sync_out) -> term2/1
  c1/1 -> adder_tree1/1(sync)
  c2/1 -> adder_tree2/1(sync)
  adder_tree1/2(dout) -> real_sum/1
  adder_tree2/2(dout) -> imag_sum/1
  real1/1 -> fir_dbl_tap1/1(a)
  imag1/1 -> fir_dbl_tap1/2(b)
  real_back4/1 -> fir_dbl_tap1/3(c)
  imag_back4/1 -> fir_dbl_tap1/4(d)
  fir_dbl_tap1/1(a_out) -> real_out1/1
  fir_dbl_tap1/2(b_out) -> imag_out1/1
  fir_dbl_tap1/3(c_out) -> real_back_out4/1
  fir_dbl_tap1/4(d_out) -> imag_back_out4/1
  fir_dbl_tap1/5(real) -> adder_tree1/2(din1)
  fir_dbl_tap1/6(imag) -> adder_tree2/2(din1)
  real2/1 -> fir_dbl_tap2/1(a)
  imag2/1 -> fir_dbl_tap2/2(b)
  real_back3/1 -> fir_dbl_tap2/3(c)
  imag_back3/1 -> fir_dbl_tap2/4(d)
  fir_dbl_tap2/1(a_out) -> real_out2/1
  fir_dbl_tap2/2(b_out) -> imag_out2/1
  fir_dbl_tap2/3(c_out) -> real_back_out3/1
  fir_dbl_tap2/4(d_out) -> imag_back_out3/1
  fir_dbl_tap2/5(real) -> adder_tree1/3(din2)
  fir_dbl_tap2/6(imag) -> adder_tree2/3(din2)
  real3/1 -> fir_dbl_tap3/1(a)
  imag3/1 -> fir_dbl_tap3/2(b)
  real_back2/1 -> fir_dbl_tap3/3(c)
  imag_back2/1 -> fir_dbl_tap3/4(d)
  fir_dbl_tap3/1(a_out) -> real_out3/1
  fir_dbl_tap3/2(b_out) -> imag_out3/1
  fir_dbl_tap3/3(c_out) -> real_back_out2/1
  fir_dbl_tap3/4(d_out) -> imag_back_out2/1
  fir_dbl_tap3/5(real) -> adder_tree1/4(din3)
  fir_dbl_tap3/6(imag) -> adder_tree2/4(din3)
  real4/1 -> fir_dbl_tap4/1(a)
  imag4/1 -> fir_dbl_tap4/2(b)
  real_back1/1 -> fir_dbl_tap4/3(c)
  imag_back1/1 -> fir_dbl_tap4/4(d)
  fir_dbl_tap4/1(a_out) -> real_out4/1
  fir_dbl_tap4/2(b_out) -> imag_out4/1
  fir_dbl_tap4/3(c_out) -> real_back_out1/1
  fir_dbl_tap4/4(d_out) -> imag_back_out1/1
  fir_dbl_tap4/5(real) -> adder_tree1/5(din4)
  fir_dbl_tap4/6(imag) -> adder_tree2/5(din4)

== system window_and_fft_test/dec_fir1/imag_sum ==
  sync : Inport
  din1 : Inport  Port=2
  din2 : Inport  Port=3
  addr1 : xbsIndex_r4/AddSub  mode=Addition  use_carryin=off  use_carryout=off  en=off  latency=1  precision=Full  arith_type=Unsigned  n_bits=16  bin_pt=14  quantization=Truncate  overflow=Wrap  dbl_ovrd=off  use_behavioral_HDL=off  hw_selection=DSP48  pipelined=on  use_rpm=on  block_type=addsub
  sync_delay : xbsIndex_r4/Delay  rst=off  infoeditControl=Selection of Reset will increase slice count due to use of real FFs and instead of SRLs  en=off  latency=1  dbl_ovrd=off  reg_retiming=on  block_type=delay
      settings: block_version=11.4
  sync_out : Outport
  dout : Outport  Port=2
  wires:
  sync/1 -> sync_delay/1
  sync_delay/1 -> sync_out/1
  din1/1 -> addr1/1
  din2/1 -> addr1/2
  addr1/1 -> dout/1

== system window_and_fft_test/dec_fir1/real_sum ==
  sync : Inport
  din1 : Inport  Port=2
  din2 : Inport  Port=3
  addr1 : xbsIndex_r4/AddSub  mode=Addition  use_carryin=off  use_carryout=off  en=off  latency=1  precision=Full  arith_type=Unsigned  n_bits=16  bin_pt=14  quantization=Truncate  overflow=Wrap  dbl_ovrd=off  use_behavioral_HDL=off  hw_selection=DSP48  pipelined=on  use_rpm=on  block_type=addsub
  sync_delay : xbsIndex_r4/Delay  rst=off  infoeditControl=Selection of Reset will increase slice count due to use of real FFs and instead of SRLs  en=off  latency=1  dbl_ovrd=off  reg_retiming=on  block_type=delay
      settings: block_version=11.4
  sync_out : Outport
  dout : Outport  Port=2
  wires:
  sync/1 -> sync_delay/1
  sync_delay/1 -> sync_out/1
  din1/1 -> addr1/1
  din2/1 -> addr1/2
  addr1/1 -> dout/1

== system window_and_fft_test/fft_wideband_real1/del_4x_pol0 ==
  d : Inport
  q : Outport
  wires:
  d/1 -> q/1

== system window_and_fft_test/fft_wideband_real1/del_4x_pol1 ==
  d : Inport
  q : Outport
  wires:
  d/1 -> q/1

== system window_and_fft_test/fft_wideband_real1/del_4x_pol2 ==
  d : Inport
  q : Outport
  wires:
  d/1 -> q/1

== system window_and_fft_test/fft_wideband_real1/del_4x_pol3 ==
  d : Inport
  q : Outport
  wires:
  d/1 -> q/1

== system window_and_fft_test/fft_wideband_real1/del_direct1 ==
  d : Inport
  q : Outport
  wires:
  d/1 -> q/1

== system window_and_fft_test/fft_wideband_real1/del_direct2 ==
  d : Inport
  q : Outport
  wires:
  d/1 -> q/1

== system window_and_fft_test/fft_wideband_real1/del_sync_4x ==
  d : Inport
  q : Outport
  wires:
  d/1 -> q/1

== system window_and_fft_test/fft_wideband_real1/fft_biplex_real_4x ==
  sync : Inport
  shift : Inport  Port=2
  pol0_in : Inport  Port=3
  pol1_in : Inport  Port=4
  pol2_in : Inport  Port=5
  pol3_in : Inport  Port=6
  bi_real_unscr_4x : Subsystem  AncestorBlock=casper_library_ffts_internal/bi_real_unscr_4x  mask(bi_real_unscr_4x){n_inputs=1, FFTSize=9, n_bits=18, bin_pt=17, add_latency=add_latency, conv_latency=conv_latency, bram_latency=bram_latency, bram_map=on, bram_delays=on, dsp48_adders=off, async=off}
      mask prompts: n_inputs "Number simultaneous inputs (2*?)"; FFTSize "Size of FFT (2^?):"; n_bits "Sample Bit Width"; bin_pt "Sample binary point"; add_latency "Add Latency"; conv_latency "Convert Latency"; bram_latency "BRAM Latency"; bram_map "Use BlockRAM for Map"; bram_delays "Use BlockRAM for Delays"; dsp48_adders "Use DSP48s for adders"; async "Asynchonrous operation"
      mask help: FFT internal block.
      mask init:
      | bi_real_unscr_4x_init(gcb, ...
      |     'n_inputs', n_inputs, ...
      |     'FFTSize', FFTSize, ...
      |     'n_bits', n_bits, ...
      |     'bin_pt', bin_pt, ...
      |     'add_latency', add_latency, ...
      |     'conv_latency', conv_latency, ...
      |     'bram_latency', bram_latency, ...
      |     'bram_map', bram_map, ...
      |     'bram_delays', bram_delays, ...
      |     'dsp48_adders', dsp48_adders, ...
      |     'async', async);
  biplex_core : Subsystem  AncestorBlock=casper_library_ffts/biplex_core  mask(biplex_core){n_inputs=1, FFTSize=9, input_bit_width=18, bin_pt_in=17, coeff_bit_width=18, add_latency=1, mult_latency=2, bram_latency=2, conv_latency=1, quantization=Round  (unbiased: +/- Inf), overflow=Saturate, delays_bit_limit=8, coeffs_bit_limit=9, coeff_sharing=on, coeff_decimation=on, max_fanout=4, mult_spec=[2 2 2 2 2 2 2 2 2], bitgrowth=off, max_bits=19, hardcode_shifts=off, shift_schedule=[1 1 1 1 1 1 1 1 1], dsp48_adders=off, async=off}
      mask prompts: n_inputs "Number inputs (2*?)"; FFTSize "Size of FFT: (2^? pts)"; input_bit_width "Input Bit Width"; bin_pt_in "Input binary point"; coeff_bit_width "Coefficient Bit Width"; add_latency "Add Latency"; mult_latency "Mult Latency"; bram_latency "BRAM Latency"; conv_latency "Convert latency"; quantization "Quantization Behavior"; overflow "Overflow Behavior"; delays_bit_limit "Number bits above which to implent stage's delays in BRAM (2^? bits)"; coeffs_bit_limit "Number bits above which to store stage's coefficients in BRAM (2^? bits)"; coeff_sharing "BRAM sharing in coeff storage"; coeff_decimation "Store a fraction of coeff factors where useful"; max_fanout "Maximum fanout"; mult_spec "Multiplier impl. (0=core, 1=embedded, 2=behavioural) (left=1st stage, or just one value)"; bitgrowth "Bit growth instead of shift"; max_bits "Maximum number of bits"; hardcode_shifts "Hardcode shift schedule"; shift_schedule "Shift schedule"; dsp48_adders "Use DSP48s for adders"; async "Asynchronous operation"
      mask help: FFT internal block.
      mask init:
      | biplex_core_init(gcb, ...
      |     'n_inputs', n_inputs, ...
      |     'FFTSize', FFTSize,...
      |     'input_bit_width', input_bit_width,...
      |     'bin_pt_in', bin_pt_in,...
      |     'coeff_bit_width', coeff_bit_width,...
      |     'async', async, ...
      |     'add_latency', add_latency,...
      |     'mult_latency', mult_latency,...
      |     'bram_latency', bram_latency,...
      |     'conv_latency', conv_latency, ...
      |     'quantization', quantization,...
      |     'overflow', overflow,...
      |     'delays_bit_limit', delays_bit_limit, ...
      |     'coeffs_bit_limit', coeffs_bit_limit, ...
      |     'coeff_sharing', coeff_sharing, ...
      |     'coeff_decimation', coeff_decimation, ...
      |     'max_fanout', max_fanout, ...
      |     'mult_spec', mult_spec, ...
      |     'bitgrowth', bitgrowth, ...
      |     'max_bits', max_bits, ...
      |     'hardcode_shifts', hardcode_shifts, ...
      |     'shift_schedule', shift_schedule, ...
      |     'dsp48_adders', dsp48_adders);
      settings: AttributesFormatString=9 stages
      mask TypeOptions quantization: Truncate | Round  (unbiased: +/- Inf) | Round  (unbiased: Even Values)
      mask TypeOptions overflow: Wrap | Saturate | Error
      mask Callback hardcode_shifts:
      | hardcode_shifts = get_param(gcb, 'hardcode_shifts');
      | set_param_state(gcb, 'shift_schedule', hardcode_shifts);
      mask Callback dsp48_adders: fft_callback_dsp48_adders(gcb);
  even_bussify : Subsystem  AncestorBlock=casper_library_flow_control/bus_create  mask(bus_create){inputNum=1}
      mask prompts: inputNum "Number of inputs:"
      mask init:
      | bus_create_init(gcb,...
      |     'inputNum', inputNum);
  odd_bussify : Subsystem  AncestorBlock=casper_library_flow_control/bus_create  mask(bus_create){inputNum=1}
      mask prompts: inputNum "Number of inputs:"
      mask init:
      | bus_create_init(gcb,...
      |     'inputNum', inputNum);
  pol0_debus : Subsystem  AncestorBlock=casper_library_flow_control/bus_expand  mask(bus_expand){mode=divisions of equal size, outputNum=1, outputWidth=36, outputBinaryPt=0, outputArithmeticType=0, show_format=off, outputToWorkspace=off, variablePrefix=out, outputToModelAsWell=on}
      mask prompts: outputNum "Number of outputs:"; outputWidth "Output width:"; outputBinaryPt "Output binary point position:"; outputArithmeticType "Output arithmetic type (ufix=0, fix=1, bool=2):"; show_format "Print format string?"; outputToWorkspace "Output to workspace?"; variablePrefix "Variable name prefix:"; outputToModelAsWell "Output to model as well?"
      mask help:
      | Expands a 'bus' made using a bus_create or Xilinx
      | concat block.
      | The input will be divided into the specified number
      | of outputs with the specified arithmetic types.
      | Divisions are made from most significant bit.
      mask init:
      | bus_expand_init(gcb,...
      |     'mode', mode, ...
      |     'outputNum', outputNum, ...
      |     'outputWidth', outputWidth, ...
      |     'outputBinaryPt', outputBinaryPt, ...
      |     'outputArithmeticType', outputArithmeticType, ...
      |     'show_format', show_format, ...
      |     'outputToWorkspace', outputToWorkspace, ...
      |     'variablePrefix', variablePrefix, ...
      |     'outputToModelAsWell', outputToModelAsWell);
      settings: AttributesFormatString=1 outputs
      mask TypeOptions mode: divisions of equal size | divisions of arbitrary size
      mask Callback mode: bus_expand_callback();
      mask Callback outputWidth: bus_expand_callback();
      mask Callback outputToWorkspace: bus_expand_callback();
  pol1_debus : Subsystem  AncestorBlock=casper_library_flow_control/bus_expand  mask(bus_expand){mode=divisions of equal size, outputNum=1, outputWidth=36, outputBinaryPt=0, outputArithmeticType=0, show_format=off, outputToWorkspace=off, variablePrefix=out, outputToModelAsWell=on}
      mask prompts: outputNum "Number of outputs:"; outputWidth "Output width:"; outputBinaryPt "Output binary point position:"; outputArithmeticType "Output arithmetic type (ufix=0, fix=1, bool=2):"; show_format "Print format string?"; outputToWorkspace "Output to workspace?"; variablePrefix "Variable name prefix:"; outputToModelAsWell "Output to model as well?"
      mask help:
      | Expands a 'bus' made using a bus_create or Xilinx
      | concat block.
      | The input will be divided into the specified number
      | of outputs with the specified arithmetic types.
      | Divisions are made from most significant bit.
      mask init: same as window_and_fft_test/fft_wideband_real1/fft_biplex_real_4x/pol0_debus
      settings: AttributesFormatString=1 outputs
      mask TypeOptions mode: divisions of equal size | divisions of arbitrary size
      mask Callback mode: bus_expand_callback();
      mask Callback outputWidth: bus_expand_callback();
      mask Callback outputToWorkspace: bus_expand_callback();
  pol2_debus : Subsystem  AncestorBlock=casper_library_flow_control/bus_expand  mask(bus_expand){mode=divisions of equal size, outputNum=1, outputWidth=36, outputBinaryPt=0, outputArithmeticType=0, show_format=off, outputToWorkspace=off, variablePrefix=out, outputToModelAsWell=on}
      mask prompts: outputNum "Number of outputs:"; outputWidth "Output width:"; outputBinaryPt "Output binary point position:"; outputArithmeticType "Output arithmetic type (ufix=0, fix=1, bool=2):"; show_format "Print format string?"; outputToWorkspace "Output to workspace?"; variablePrefix "Variable name prefix:"; outputToModelAsWell "Output to model as well?"
      mask help:
      | Expands a 'bus' made using a bus_create or Xilinx
      | concat block.
      | The input will be divided into the specified number
      | of outputs with the specified arithmetic types.
      | Divisions are made from most significant bit.
      mask init: same as window_and_fft_test/fft_wideband_real1/fft_biplex_real_4x/pol0_debus
      settings: AttributesFormatString=1 outputs
      mask TypeOptions mode: divisions of equal size | divisions of arbitrary size
      mask Callback mode: bus_expand_callback();
      mask Callback outputWidth: bus_expand_callback();
      mask Callback outputToWorkspace: bus_expand_callback();
  pol3_debus : Subsystem  AncestorBlock=casper_library_flow_control/bus_expand  mask(bus_expand){mode=divisions of equal size, outputNum=1, outputWidth=36, outputBinaryPt=0, outputArithmeticType=0, show_format=off, outputToWorkspace=off, variablePrefix=out, outputToModelAsWell=on}
      mask prompts: outputNum "Number of outputs:"; outputWidth "Output width:"; outputBinaryPt "Output binary point position:"; outputArithmeticType "Output arithmetic type (ufix=0, fix=1, bool=2):"; show_format "Print format string?"; outputToWorkspace "Output to workspace?"; variablePrefix "Variable name prefix:"; outputToModelAsWell "Output to model as well?"
      mask help:
      | Expands a 'bus' made using a bus_create or Xilinx
      | concat block.
      | The input will be divided into the specified number
      | of outputs with the specified arithmetic types.
      | Divisions are made from most significant bit.
      mask init: same as window_and_fft_test/fft_wideband_real1/fft_biplex_real_4x/pol0_debus
      settings: AttributesFormatString=1 outputs
      mask TypeOptions mode: divisions of equal size | divisions of arbitrary size
      mask Callback mode: bus_expand_callback();
      mask Callback outputWidth: bus_expand_callback();
      mask Callback outputToWorkspace: bus_expand_callback();
  ri_to_c0 : Subsystem  AncestorBlock=casper_library_misc/ri_to_c  mask(ri_to_c){}
      mask help:
      | Concatenates real and imaginary inputs into a complex output.
      | Useful for simplifying interconnects.
      | See also: Complex to Real-Imag (c_to_ri)
      mask Help: eval('xlWeb(''http://casper.berkeley.edu/wiki/Ri_to_c'')')
  ri_to_c1 : Subsystem  AncestorBlock=casper_library_misc/ri_to_c  mask(ri_to_c){}
      mask help:
      | Concatenates real and imaginary inputs into a complex output.
      | Useful for simplifying interconnects.
      | See also: Complex to Real-Imag (c_to_ri)
      mask Help: eval('xlWeb(''http://casper.berkeley.edu/wiki/Ri_to_c'')')
  sync_out : Outport
  pol0_out : Outport  Port=2
  pol1_out : Outport  Port=3
  pol2_out : Outport  Port=4
  pol3_out : Outport  Port=5
  of : Outport  Port=6
  wires:
  pol0_debus/1(msb_lsb_out1) -> pol0_out/1
  pol0_in/1 -> ri_to_c0/1(re)
  pol1_in/1 -> ri_to_c0/2(im)
  ri_to_c0/1(c) -> even_bussify/1(in1)
  pol1_debus/1(msb_lsb_out1) -> pol1_out/1
  pol2_debus/1(msb_lsb_out1) -> pol2_out/1
  pol2_in/1 -> ri_to_c1/1(re)
  pol3_in/1 -> ri_to_c1/2(im)
  ri_to_c1/1(c) -> odd_bussify/1(in1)
  pol3_debus/1(msb_lsb_out1) -> pol3_out/1
  sync/1 -> biplex_core/1(sync)
  shift/1 -> biplex_core/2(shift)
  even_bussify/1(bus_out) -> biplex_core/3(pol1)
  odd_bussify/1(bus_out) -> biplex_core/4(pol2)
  biplex_core/4(of) -> of/1
  biplex_core/1(sync_out) -> bi_real_unscr_4x/1(sync)
  biplex_core/2(out1) -> bi_real_unscr_4x/2(even)
  biplex_core/3(out2) -> bi_real_unscr_4x/3(odd)
  bi_real_unscr_4x/1(sync_out) -> sync_out/1
  bi_real_unscr_4x/2(pol1_out) -> pol0_debus/1(bus_in)
  bi_real_unscr_4x/3(pol2_out) -> pol1_debus/1(bus_in)
  bi_real_unscr_4x/4(pol3_out) -> pol2_debus/1(bus_in)
  bi_real_unscr_4x/5(pol4_out) -> pol3_debus/1(bus_in)
